simulink library "Copter_Library"  (Simulink 7.3)
settings: Solver=ode45  StartTime=0.0  StopTime=10.0  RelTol=1e-3
undefined symbols (not defined in the file or in its folder): boom, f1, f2, f3, f4, f5, g, I_x, I_y, I_z, m, speed, thrust, Ts
libraries: Copter_Library x10, dspinverses x2
settings Model: Creator=robert  LastModifiedBy=Alex

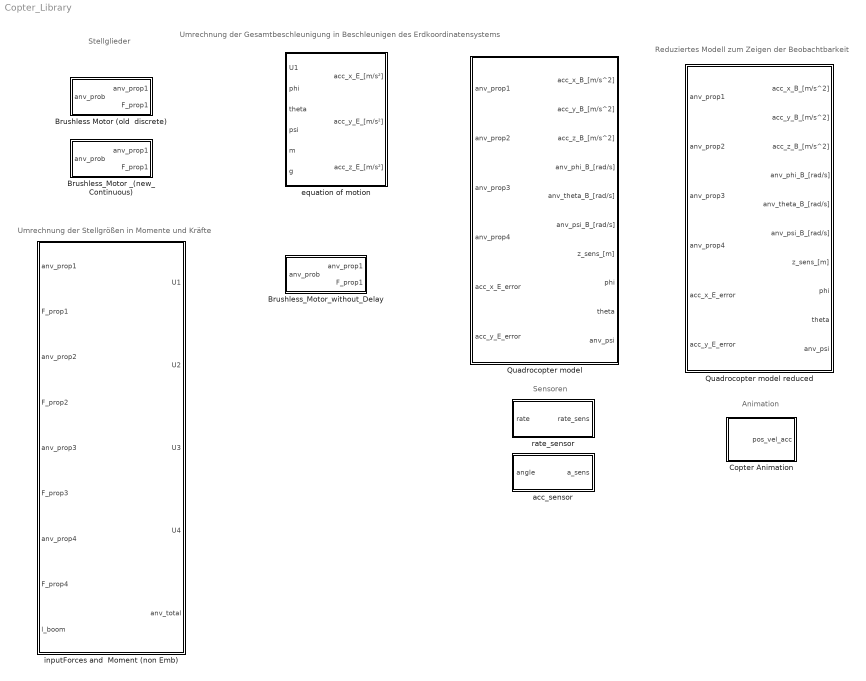
== system Copter_Library ==
  note: Sensoren
  note: Animation
  note: Umrechnung der Gesamtbeschleunigung in
      | Beschleunigen des Erdkoordinatensystems
  note: Stellglieder
  note: Umrechnung der Stellgrößen
      | in Momente und Kräfte
  note: Reduziertes Modell zum Zeigen der
      | Beobachtbarkeit
  Brushless Motor (old  discrete) : Subsystem
  Brushless_Motor _(new_Continuous) : Subsystem  mask{M_error=0.99}
      mask prompts: M_error "Motor-Force pitch error [1 = no error, 0.9 = 10% negativ error, 1.1 = 10% positive error]:"
  Brushless_Motor_without_Delay : Subsystem  AncestorBlock=Copter_Library/Brushless_Motor _(new_Continuous)  mask{M_error=0.99}
      mask prompts: M_error "Motor-Force pitch error [1 = no error, 0.9 = 10% negativ error, 1.1 = 10% positive error]:"
  Copter Animation : Subsystem  mask(Quadrocopter Animation){AXES=[-100 100 -100 100 0 100], T_INT=1/25, K_VAR=Feste Position, K_POS=[10 0 2], K_ANGLE=27, A_ON=on, u_phi=on, u_theta=on, u_psi=on, u_x=on, u_y=on, u_z=off}
      mask prompts: AXES "Achsen Grenzen [xmin xmax ymin ymax zmin zmax]"; T_INT "Zeitintervall zwischen Aktualisierungen [s]:"; K_VAR "Kamera Art:"; K_POS "Ort der Kamera [xc yc zc]:"; K_ANGLE "Öffnungswinkel der Kamera [Grad]:"; A_ON "Animation Einschalten:"; u_phi "Use Input phi:"; u_theta "Use Input theta:"; u_psi "Use Input psi:"; u_x "Use Input x:"; u_y "Use Input y:"; u_z "Use Input z:"
      mask help: Erstellt eine 3-D animierte Ansicht eines Quadrocopters.
      mask init:
      | Config.axes = AXES;
      | Config.update = T_INT;
      | Config.camera_view = K_VAR;
      | Config.camera_pos = K_POS;
      | Config.view = K_ANGLE;
      | Config.Animenable = A_ON;
      | Config.phi = u_phi;
      | Config.theta = u_theta;
      | Config.psi = u_psi;
      | Config.x = u_x;
      | Config.y = u_y;
      | Config.z = u_z;
      mask Help:
      | <p>Dieser Block erstellt ein 3 dimensionales Fenster eines Quadrocopters.
      | 
      | <p><H4>Block Eingänge</H4>
      | Der Eingangsvektor bestehend aus:
      | <ul>
      | <li>X-Koordinate - Ort bezogen auf die X-Achse
      | <li>Y-Koordinate - Ort bezogen auf die Y-Achse
      | <li>Z-Koordinate - Ort bezogen auf die Z-Achse
      | <li>Psi - Yaw Drehung um die Z-Achse
      | <li>Phi - Roll Drehen um die Achse in Flugrichtung
      | <li>theta - pitch Neigung in Flugrichtung nach oben bzw. unten
      | </ul></p>
      mask StyleString: edit,edit,popup(Feste Position|Frei bewegbar),edit,edit,checkbox,checkbox,checkbox,checkbox,checkbox,checkbox,checkbox
  Quadrocopter model : Subsystem
  Quadrocopter model reduced : Subsystem
  acc_sensor : Subsystem  mask{lsb_per_g=g/340, direction=1}
      mask prompts: lsb_per_g "Auflösung[LSB/g]:(g = Erdbeschleunigung)"; direction "Direction[-1 ... 1]:"
      mask init:
      | LSB_per_g = lsb_per_g;
      | Direction = direction;
  equation of motion : Subsystem
  inputForces and  Moment (non Emb) : Subsystem
  rate_sensor : Subsystem  mask{resolution=0.01423597337917052316100312926969, offset=505, direction=1}
      mask prompts: resolution "Resolution [(rad/sec)/LSB)]:"; offset "Offset [LSB]:"; direction "Direction [-1 ... 1]"
      mask init:
      | Resolution = resolution;
      | Offset = offset;
      | Direction = direction;

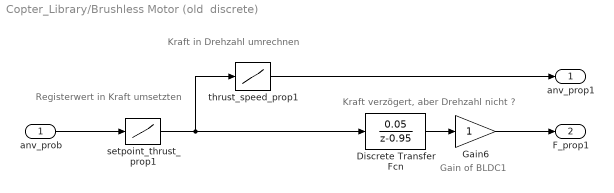
== system Copter_Library/Brushless Motor (old  discrete) ==
  note: Gain of BLDC1
  note: Kraft in Drehzahl umrechnen
  note: Registerwert in Kraft umsetzten
  note: Kraft verzögert, aber Drehzahl nicht ?
  anv_prob : Inport  OutDataType=fixdt(1, 16)  OutScaling=2^0
  Discrete Transfer Fcn : DiscreteTransferFcn  Numerator=[0.05]  Denominator=[1 -0.95]  SampleTime=Ts
  Gain6 : Gain  ParameterDataType=fixdt(1, 16)  ParameterScaling=2^0  OutDataType=fixdt(1, 16)  OutScaling=2^0
  setpoint_thrust_prop1 : Lookup  InputValues=[0 40 175]  Table=[0 500 4500]./1000  LookUpMeth=Interpolation-Use End Values  OutDataType=fixdt(1, 16)  OutScaling=2^0
  thrust_speed_prop1 : Lookup  InputValues=thrust  Table=speed  LookUpMeth=Interpolation-Use End Values  OutDataType=fixdt(1, 16)  OutScaling=2^0
  anv_prop1 : Outport  OutDataType=fixdt(1, 16)  OutScaling=2^0
  F_prop1 : Outport  Port=2  OutDataType=fixdt(1, 16)  OutScaling=2^0
  wires:
  anv_prob/1 -> setpoint_thrust_prop1/1
  Discrete Transfer Fcn/1 -> Gain6/1
  Gain6/1 -> F_prop1/1
  thrust_speed_prop1/1 -> anv_prop1/1
  setpoint_thrust_prop1/1 -> thrust_speed_prop1/1, Discrete Transfer Fcn/1

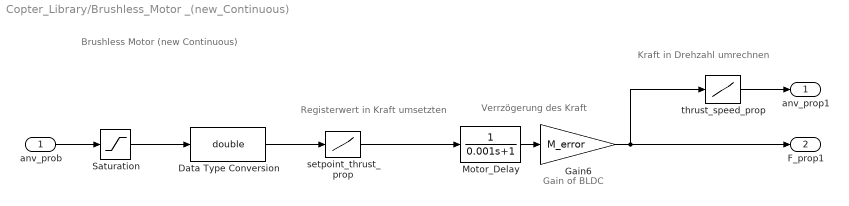
== system Copter_Library/Brushless_Motor _(new_Continuous) ==
  note: Gain of BLDC
  note: Kraft in Drehzahl umrechnen
  note: Registerwert in Kraft umsetzten
  note: Verrzögerung des Kraft
  note: Brushless Motor (new Continuous)
  anv_prob : Inport  OutDataType=fixdt(1, 16)  OutScaling=2^0
  Data Type Conversion : DataTypeConversion  OutDataTypeMode=double  OutDataType=fixdt(1, 16)  OutScaling=2^0  OutDataTypeStr=double
  Gain6 : Gain  Gain=M_error  ParameterDataType=fixdt(1, 16)  ParameterScaling=2^0  OutDataType=fixdt(1, 16)  OutScaling=2^0
  Motor_Delay : TransferFcn  Denominator=[0.001 1]  ContinuousStateAttributes='Motor_Delay'
  Saturation : Saturate  UpperLimit=255  LowerLimit=0  OutDataType=fixdt(1, 16)  OutScaling=2^0
  setpoint_thrust_prop : Lookup  InputValues=[0 40 175]  Table=[0 500 4500]./1000  LookUpMeth=Interpolation-Use End Values  OutDataType=fixdt(1, 16)  OutScaling=2^0
  thrust_speed_prop : Lookup  InputValues=thrust  Table=speed  LookUpMeth=Interpolation-Use End Values  OutDataType=fixdt(1, 16)  OutScaling=2^0
  anv_prop1 : Outport  OutDataType=fixdt(1, 16)  OutScaling=2^0
  F_prop1 : Outport  Port=2  OutDataType=fixdt(1, 16)  OutScaling=2^0
  wires:
  setpoint_thrust_prop/1 -> Motor_Delay/1
  Saturation/1 -> Data Type Conversion/1
  anv_prob/1 -> Saturation/1
  Data Type Conversion/1 -> setpoint_thrust_prop/1
  Motor_Delay/1 -> Gain6/1
  Gain6/1 -> F_prop1/1, thrust_speed_prop/1
  thrust_speed_prop/1 -> anv_prop1/1

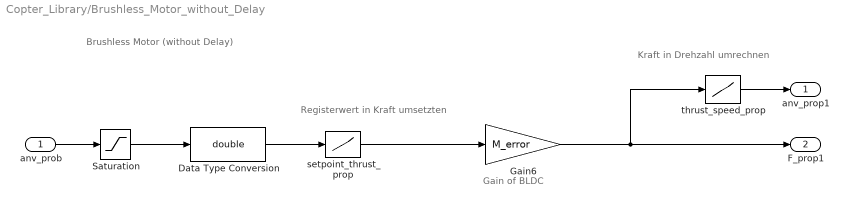
== system Copter_Library/Brushless_Motor_without_Delay ==
  note: Gain of BLDC
  note: Kraft in Drehzahl umrechnen
  note: Registerwert in Kraft umsetzten
  note: Brushless Motor (without Delay)
  anv_prob : Inport  OutDataType=fixdt(1, 16)  OutScaling=2^0
  Data Type Conversion : DataTypeConversion  OutDataTypeMode=double  OutDataType=fixdt(1, 16)  OutScaling=2^0  OutDataTypeStr=double
  Gain6 : Gain  Gain=M_error  ParameterDataType=fixdt(1, 16)  ParameterScaling=2^0  OutDataType=fixdt(1, 16)  OutScaling=2^0
  Saturation : Saturate  UpperLimit=255  LowerLimit=0  OutDataType=fixdt(1, 16)  OutScaling=2^0
  setpoint_thrust_prop : Lookup  InputValues=[0 40 175]  Table=[0 500 4500]./1000  LookUpMeth=Interpolation-Use End Values  OutDataType=fixdt(1, 16)  OutScaling=2^0
  thrust_speed_prop : Lookup  InputValues=thrust  Table=speed  LookUpMeth=Interpolation-Use End Values  OutDataType=fixdt(1, 16)  OutScaling=2^0
  anv_prop1 : Outport  OutDataType=fixdt(1, 16)  OutScaling=2^0
  F_prop1 : Outport  Port=2  OutDataType=fixdt(1, 16)  OutScaling=2^0
  wires:
  setpoint_thrust_prop/1 -> Gain6/1
  Saturation/1 -> Data Type Conversion/1
  anv_prob/1 -> Saturation/1
  Data Type Conversion/1 -> setpoint_thrust_prop/1
  Gain6/1 -> F_prop1/1, thrust_speed_prop/1
  thrust_speed_prop/1 -> anv_prop1/1

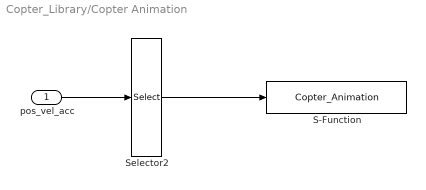
== system Copter_Library/Copter Animation ==
  pos_vel_acc : Inport  PortDimensions=19  OutDataType=sfix(16)  OutScaling=2^0
  S-Function : S-Function  FunctionName=Copter_Animation  Parameters=Config  EnableBusSupport=off
  Selector2 : Selector  InputPortWidth=19  IndexOptions=Index vector (dialog)  Indices=[1 2 3 4 5 6]  OutputSizes=1
  wires:
  Selector2/1 -> S-Function/1
  pos_vel_acc/1 -> Selector2/1

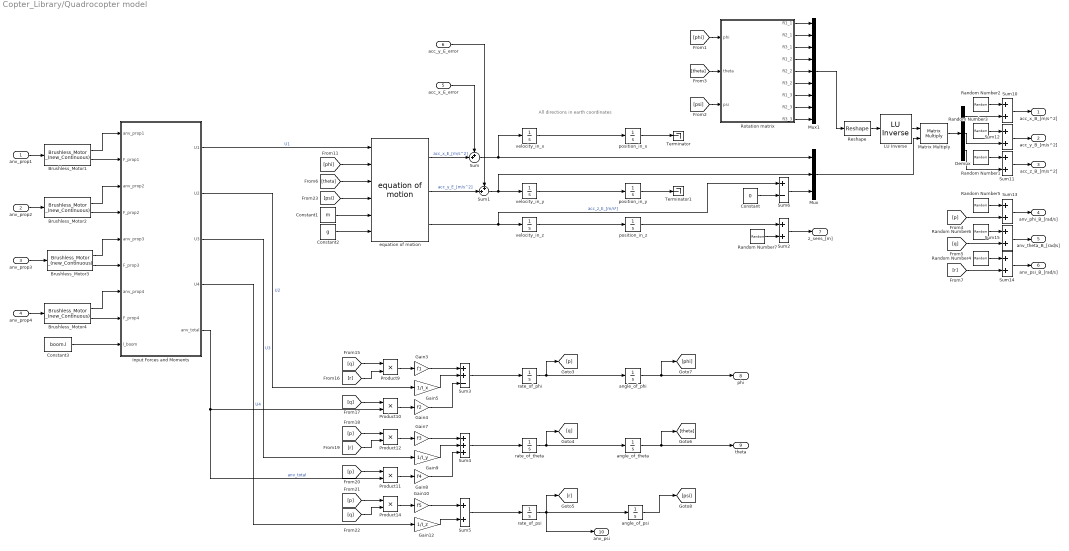
== system Copter_Library/Quadrocopter model ==
  note: All directions in earth coordinates
  anv_prop1 : Inport  OutDataType=fixdt(1, 16)  OutScaling=2^0
  anv_prop2 : Inport  Port=2  OutDataType=fixdt(1, 16)  OutScaling=2^0
  anv_prop3 : Inport  Port=3  OutDataType=fixdt(1, 16)  OutScaling=2^0
  anv_prop4 : Inport  Port=4  OutDataType=fixdt(1, 16)  OutScaling=2^0
  acc_x_E_error : Inport  Port=5  OutDataType=fixdt(1, 16)  OutScaling=2^0
  acc_y_E_error : Inport  Port=6  OutDataType=fixdt(1, 16)  OutScaling=2^0
  " LU Inverse" : dspinverses/ LU Inverse  SystemSampleTime=-1
  Brushless_Motor{1..4} (4 alike) : Copter_Library/Brushless_Motor _(new_Continuous)  SystemSampleTime=-1
  Constant : Constant  Value=0  OutDataType=fixdt(1, 16)  OutScaling=2^0  SampleTime=Ts
  Constant1 : Constant  Value=m  OutDataType=fixdt(1, 16)  OutScaling=2^0  SampleTime=Ts
  Constant2 : Constant  Value=g  OutDataType=fixdt(1, 16)  OutScaling=2^0  SampleTime=Ts
  Constant3 : Constant  Value=boom.l  OutDataType=fixdt(1, 16)  OutScaling=2^0
  Demux : Demux  Outputs=3
  Gain10 : Gain  Gain=f5  ParameterDataType=fixdt(1, 16)  ParameterScaling=2^0  OutDataType=fixdt(1, 16)  OutScaling=2^0
  Gain12 : Gain  Gain=1/I_z  ParameterDataType=fixdt(1, 16)  ParameterScaling=2^0  OutDataType=fixdt(1, 16)  OutScaling=2^0
  Gain3 : Gain  Gain=f1  ParameterDataType=fixdt(1, 16)  ParameterScaling=2^0  OutDataType=fixdt(1, 16)  OutScaling=2^0
  Gain4 : Gain  Gain=f2  ParameterDataType=fixdt(1, 16)  ParameterScaling=2^0  OutDataType=fixdt(1, 16)  OutScaling=2^0
  Gain5 : Gain  Gain=1/I_x  ParameterDataType=fixdt(1, 16)  ParameterScaling=2^0  OutDataType=fixdt(1, 16)  OutScaling=2^0
  Gain7 : Gain  Gain=f3  ParameterDataType=fixdt(1, 16)  ParameterScaling=2^0  OutDataType=fixdt(1, 16)  OutScaling=2^0
  Gain8 : Gain  Gain=f4  ParameterDataType=fixdt(1, 16)  ParameterScaling=2^0  OutDataType=fixdt(1, 16)  OutScaling=2^0
  Gain9 : Gain  Gain=1/I_y  ParameterDataType=fixdt(1, 16)  ParameterScaling=2^0  OutDataType=fixdt(1, 16)  OutScaling=2^0
  Input Forces and Moments : Stateflow chart
  Matrix Multiply : Product  Multiplication=Matrix(*)  OutDataType=sfix(16)  OutScaling=2^0
  Mux : Mux  Inputs=3
  Mux1 : Mux  Inputs=9
  Product{9..12,14} (5 alike) : Product  OutDataType=fixdt(1, 16)  OutScaling=2^0  RndMeth=Zero
  Random Number{1..7} (7 alike) : RandomNumber  Variance=0  SampleTime=Ts
  Reshape : Reshape  OutputDimensionality=Customize  OutputDimensions=[3,3]
  Rotation matrix : Stateflow chart
  Sum : Sum  Inputs=++|  OutDataType=fixdt(1, 16)  OutScaling=2^0
  Sum1 : Sum  Inputs=++|  OutDataType=fixdt(1, 16)  OutScaling=2^0
  Sum{2,5,10..15} (8 alike) : Sum  OutDataType=fixdt(1, 16)  OutScaling=2^0
  Sum3 : Sum  Inputs=++-  OutDataType=fixdt(1, 16)  OutScaling=2^0
  Sum4 : Sum  Inputs=+++  OutDataType=fixdt(1, 16)  OutScaling=2^0
  Sum6 : Sum  Inputs=+-  OutDataType=fixdt(1, 16)  OutScaling=2^0
  Terminator : Terminator
  Terminator1 : Terminator
  angle_of_phi : Integrator
  angle_of_psi : Integrator
  angle_of_theta : Integrator
  equation of motion : Copter_Library/equation of motion  SystemSampleTime=-1
  position_in_x : Integrator
  position_in_y : Integrator
  position_in_z : Integrator
  rate_of_phi : Integrator
  rate_of_psi : Integrator
  rate_of_theta : Integrator
  velocity_in_x : Integrator
  velocity_in_y : Integrator
  velocity_in_z : Integrator
  acc_x_B_[m/s^2] : Outport  OutDataType=fixdt(1, 16)  OutScaling=2^0
  acc_y_B_[m/s^2] : Outport  Port=2  OutDataType=fixdt(1, 16)  OutScaling=2^0
  acc_z_B_[m/s^2] : Outport  Port=3  OutDataType=fixdt(1, 16)  OutScaling=2^0
  anv_phi_B_[rad/s] : Outport  Port=4  OutDataType=fixdt(1, 16)  OutScaling=2^0
  anv_theta_B_[rad/s] : Outport  Port=5  OutDataType=fixdt(1, 16)  OutScaling=2^0
  anv_psi_B_[rad/s] : Outport  Port=6  OutDataType=fixdt(1, 16)  OutScaling=2^0
  z_sens_[m] : Outport  Port=7  OutDataType=fixdt(1, 16)  OutScaling=2^0
  phi : Outport  Port=8  OutDataType=fixdt(1, 16)  OutScaling=2^0
  theta : Outport  Port=9  OutDataType=fixdt(1, 16)  OutScaling=2^0
  anv_psi : Outport  Port=10  OutDataType=fixdt(1, 16)  OutScaling=2^0
  wires:
  Sum14/1 -> anv_psi_B_[rad/s]/1
  Sum15/1 -> anv_theta_B_[rad/s]/1
  Sum13/1 -> anv_phi_B_[rad/s]/1
  [q] -> Sum15/2
  Random Number6/1 -> Sum15/1
  [r] -> Sum14/2
  Random Number4/1 -> Sum14/1
  [p] -> Sum13/2
  Random Number5/1 -> Sum13/1
  Sum11/1 -> acc_z_B_[m/s^2]/1
  Sum12/1 -> acc_y_B_[m/s^2]/1
  Sum10/1 -> acc_x_B_[m/s^2]/1
  Demux/2 -> Sum12/2
  Random Number3/1 -> Sum12/1
  Demux/3 -> Sum11/2
  Random Number1/1 -> Sum11/1
  Demux/1 -> Sum10/2
  Random Number2/1 -> Sum10/1
  Matrix Multiply/1 -> Demux/1
  anv_prop3/1 -> Brushless_Motor3/1
  anv_prop4/1 -> Brushless_Motor4/1
  Reshape/1 -> " LU Inverse"/1
  Mux/1 -> Matrix Multiply/2
  Mux1/1 -> Reshape/1
  Rotation matrix/9(R3_3) -> Mux1/9
  Rotation matrix/8(R2_3) -> Mux1/8
  Rotation matrix/7(R1_3) -> Mux1/7
  Rotation matrix/6(R3_2) -> Mux1/6
  Rotation matrix/5(R2_2) -> Mux1/5
  Rotation matrix/4(R1_2) -> Mux1/4
  Rotation matrix/3(R3_1) -> Mux1/3
  Rotation matrix/2(R2_1) -> Mux1/2
  Rotation matrix/1(R1_1) -> Mux1/1
  [psi] -> Rotation matrix/3(psi)
  [theta] -> Rotation matrix/2(theta)
  [phi] -> Rotation matrix/1(phi)
  anv_prop2/1 -> Brushless_Motor2/1
  anv_prop1/1 -> Brushless_Motor1/1
  velocity_in_x/1 -> position_in_x/1
  velocity_in_y/1 -> position_in_y/1
  velocity_in_z/1 -> position_in_z/1
  Constant3/1 -> Input Forces and Moments/9(l_boom)
  Sum5/1 -> rate_of_psi/1
  Input Forces and Moments/4(U4) -> Gain12/1  "U4"
  Gain12/1 -> Sum5/2
  Gain10/1 -> Sum5/1
  Product14/1 -> Gain10/1
  [q] -> Product14/2
  [p] -> Product14/1
  Sum4/1 -> rate_of_theta/1
  Input Forces and Moments/3(U3) -> Gain9/1  "U3"
  Gain8/1 -> Sum4/3
  Gain9/1 -> Sum4/2
  Product11/1 -> Gain8/1
  [p] -> Product11/1
  Gain7/1 -> Sum4/1
  Product12/1 -> Gain7/1
  [r] -> Product12/2
  [p] -> Product12/1
  Input Forces and Moments/1(U1) -> equation of motion/1  "U1"
  Sum3/1 -> rate_of_phi/1
  Gain4/1 -> Sum3/3
  Gain5/1 -> Sum3/2
  Input Forces and Moments/2(U2) -> Gain5/1  "U2"
  Product10/1 -> Gain4/1
  [q] -> Product10/1
  Gain3/1 -> Sum3/1
  Product9/1 -> Gain3/1
  [r] -> Product9/2
  [q] -> Product9/1
  Input Forces and Moments/5(anv_total) -> Product11/2, Product10/2  "anv_total"
  angle_of_phi/1 -> [phi], phi/1
  angle_of_theta/1 -> [theta], theta/1
  angle_of_psi/1 -> [psi]
  rate_of_phi/1 -> [p], angle_of_phi/1
  rate_of_theta/1 -> angle_of_theta/1, [q]
  rate_of_psi/1 -> anv_psi/1, angle_of_psi/1, [r]
  Constant/1 -> Sum6/2
  Sum6/1 -> Mux/3
  " LU Inverse"/1 -> Matrix Multiply/1
  Brushless_Motor1/1 -> Input Forces and Moments/1(anv_prop1)
  Brushless_Motor1/2 -> Input Forces and Moments/2(F_prop1)
  Brushless_Motor2/1 -> Input Forces and Moments/3(anv_prop2)
  Brushless_Motor2/2 -> Input Forces and Moments/4(F_prop2)
  Brushless_Motor3/1 -> Input Forces and Moments/5(anv_prop3)
  Brushless_Motor3/2 -> Input Forces and Moments/6(F_prop3)
  Brushless_Motor4/1 -> Input Forces and Moments/7(anv_prop4)
  Brushless_Motor4/2 -> Input Forces and Moments/8(F_prop4)
  [phi] -> equation of motion/2
  [theta] -> equation of motion/3
  [psi] -> equation of motion/4
  Constant1/1 -> equation of motion/5
  Constant2/1 -> equation of motion/6
  equation of motion/3 -> velocity_in_z/1, Sum6/1  "acc_z_E_[m/s²]"
  position_in_x/1 -> Terminator/1
  position_in_y/1 -> Terminator1/1
  Sum1/1 -> velocity_in_y/1, Mux/2
  equation of motion/2 -> Sum1/2  "acc_y_E_[m/s^2]"
  equation of motion/1 -> Sum/2  "acc_x_E_[m/s^2]"
  Sum/1 -> Mux/1, velocity_in_x/1
  acc_x_E_error/1 -> Sum/1
  acc_y_E_error/1 -> Sum1/1
  position_in_z/1 -> Sum2/1
  Sum2/1 -> z_sens_[m]/1
  Random Number7/1 -> Sum2/2

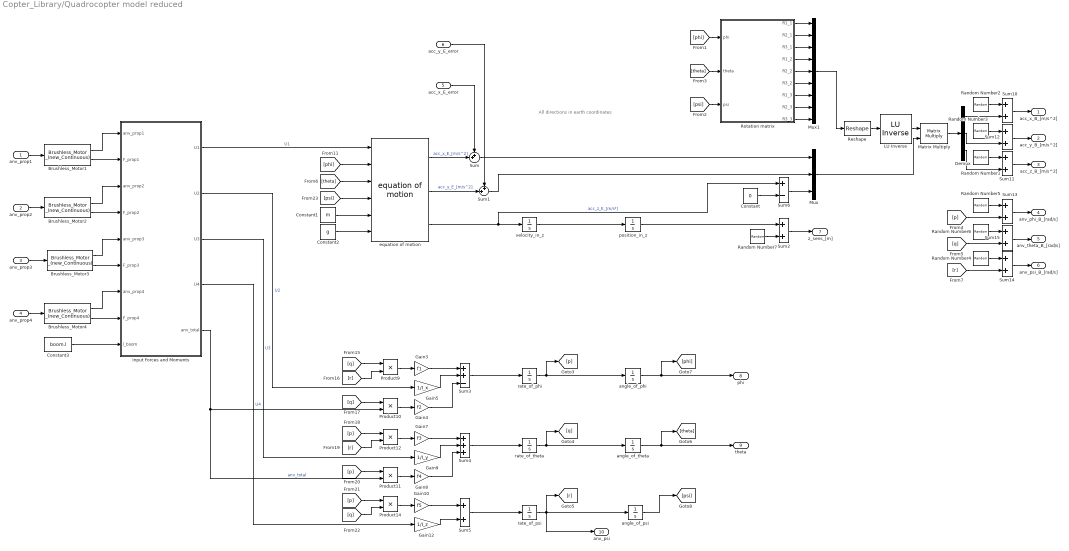
== system Copter_Library/Quadrocopter model reduced ==
  note: All directions in earth coordinates
  anv_prop1 : Inport  OutDataType=fixdt(1, 16)  OutScaling=2^0
  anv_prop2 : Inport  Port=2  OutDataType=fixdt(1, 16)  OutScaling=2^0
  anv_prop3 : Inport  Port=3  OutDataType=fixdt(1, 16)  OutScaling=2^0
  anv_prop4 : Inport  Port=4  OutDataType=fixdt(1, 16)  OutScaling=2^0
  acc_x_E_error : Inport  Port=5  OutDataType=fixdt(1, 16)  OutScaling=2^0
  acc_y_E_error : Inport  Port=6  OutDataType=fixdt(1, 16)  OutScaling=2^0
  " LU Inverse" : dspinverses/ LU Inverse  SystemSampleTime=-1
  Brushless_Motor{1..4} (4 alike) : Copter_Library/Brushless_Motor _(new_Continuous)  SystemSampleTime=-1
  Constant : Constant  Value=0  OutDataType=fixdt(1, 16)  OutScaling=2^0  SampleTime=Ts
  Constant1 : Constant  Value=m  OutDataType=fixdt(1, 16)  OutScaling=2^0  SampleTime=Ts
  Constant2 : Constant  Value=g  OutDataType=fixdt(1, 16)  OutScaling=2^0  SampleTime=Ts
  Constant3 : Constant  Value=boom.l  OutDataType=fixdt(1, 16)  OutScaling=2^0
  Demux : Demux  Outputs=3
  Gain10 : Gain  Gain=f5  ParameterDataType=fixdt(1, 16)  ParameterScaling=2^0  OutDataType=fixdt(1, 16)  OutScaling=2^0
  Gain12 : Gain  Gain=1/I_z  ParameterDataType=fixdt(1, 16)  ParameterScaling=2^0  OutDataType=fixdt(1, 16)  OutScaling=2^0
  Gain3 : Gain  Gain=f1  ParameterDataType=fixdt(1, 16)  ParameterScaling=2^0  OutDataType=fixdt(1, 16)  OutScaling=2^0
  Gain4 : Gain  Gain=f2  ParameterDataType=fixdt(1, 16)  ParameterScaling=2^0  OutDataType=fixdt(1, 16)  OutScaling=2^0
  Gain5 : Gain  Gain=1/I_x  ParameterDataType=fixdt(1, 16)  ParameterScaling=2^0  OutDataType=fixdt(1, 16)  OutScaling=2^0
  Gain7 : Gain  Gain=f3  ParameterDataType=fixdt(1, 16)  ParameterScaling=2^0  OutDataType=fixdt(1, 16)  OutScaling=2^0
  Gain8 : Gain  Gain=f4  ParameterDataType=fixdt(1, 16)  ParameterScaling=2^0  OutDataType=fixdt(1, 16)  OutScaling=2^0
  Gain9 : Gain  Gain=1/I_y  ParameterDataType=fixdt(1, 16)  ParameterScaling=2^0  OutDataType=fixdt(1, 16)  OutScaling=2^0
  Input Forces and Moments : Stateflow chart
  Matrix Multiply : Product  Multiplication=Matrix(*)  OutDataType=sfix(16)  OutScaling=2^0
  Mux : Mux  Inputs=3
  Mux1 : Mux  Inputs=9
  Product{9..12,14} (5 alike) : Product  OutDataType=fixdt(1, 16)  OutScaling=2^0  RndMeth=Zero
  Random Number{1..7} (7 alike) : RandomNumber  Variance=0  SampleTime=Ts
  Reshape : Reshape  OutputDimensionality=Customize  OutputDimensions=[3,3]
  Rotation matrix : Stateflow chart
  Sum : Sum  Inputs=++|  OutDataType=fixdt(1, 16)  OutScaling=2^0
  Sum1 : Sum  Inputs=++|  OutDataType=fixdt(1, 16)  OutScaling=2^0
  Sum{2,5,10..15} (8 alike) : Sum  OutDataType=fixdt(1, 16)  OutScaling=2^0
  Sum3 : Sum  Inputs=++-  OutDataType=fixdt(1, 16)  OutScaling=2^0
  Sum4 : Sum  Inputs=+++  OutDataType=fixdt(1, 16)  OutScaling=2^0
  Sum6 : Sum  Inputs=+-  OutDataType=fixdt(1, 16)  OutScaling=2^0
  angle_of_phi : Integrator
  angle_of_psi : Integrator
  angle_of_theta : Integrator
  equation of motion : Copter_Library/equation of motion  SystemSampleTime=-1
  position_in_z : Integrator
  rate_of_phi : Integrator
  rate_of_psi : Integrator
  rate_of_theta : Integrator
  velocity_in_z : Integrator
  acc_x_B_[m/s^2] : Outport  OutDataType=fixdt(1, 16)  OutScaling=2^0
  acc_y_B_[m/s^2] : Outport  Port=2  OutDataType=fixdt(1, 16)  OutScaling=2^0
  acc_z_B_[m/s^2] : Outport  Port=3  OutDataType=fixdt(1, 16)  OutScaling=2^0
  anv_phi_B_[rad/s] : Outport  Port=4  OutDataType=fixdt(1, 16)  OutScaling=2^0
  anv_theta_B_[rad/s] : Outport  Port=5  OutDataType=fixdt(1, 16)  OutScaling=2^0
  anv_psi_B_[rad/s] : Outport  Port=6  OutDataType=fixdt(1, 16)  OutScaling=2^0
  z_sens_[m] : Outport  Port=7  OutDataType=fixdt(1, 16)  OutScaling=2^0
  phi : Outport  Port=8  OutDataType=fixdt(1, 16)  OutScaling=2^0
  theta : Outport  Port=9  OutDataType=fixdt(1, 16)  OutScaling=2^0
  anv_psi : Outport  Port=10  OutDataType=fixdt(1, 16)  OutScaling=2^0
  wires:
  Sum14/1 -> anv_psi_B_[rad/s]/1
  Sum15/1 -> anv_theta_B_[rad/s]/1
  Sum13/1 -> anv_phi_B_[rad/s]/1
  [q] -> Sum15/2
  Random Number6/1 -> Sum15/1
  [r] -> Sum14/2
  Random Number4/1 -> Sum14/1
  [p] -> Sum13/2
  Random Number5/1 -> Sum13/1
  Sum11/1 -> acc_z_B_[m/s^2]/1
  Sum12/1 -> acc_y_B_[m/s^2]/1
  Sum10/1 -> acc_x_B_[m/s^2]/1
  Demux/2 -> Sum12/2
  Random Number3/1 -> Sum12/1
  Demux/3 -> Sum11/2
  Random Number1/1 -> Sum11/1
  Demux/1 -> Sum10/2
  Random Number2/1 -> Sum10/1
  Matrix Multiply/1 -> Demux/1
  anv_prop3/1 -> Brushless_Motor3/1
  anv_prop4/1 -> Brushless_Motor4/1
  Reshape/1 -> " LU Inverse"/1
  Mux/1 -> Matrix Multiply/2
  Mux1/1 -> Reshape/1
  Rotation matrix/9(R3_3) -> Mux1/9
  Rotation matrix/8(R2_3) -> Mux1/8
  Rotation matrix/7(R1_3) -> Mux1/7
  Rotation matrix/6(R3_2) -> Mux1/6
  Rotation matrix/5(R2_2) -> Mux1/5
  Rotation matrix/4(R1_2) -> Mux1/4
  Rotation matrix/3(R3_1) -> Mux1/3
  Rotation matrix/2(R2_1) -> Mux1/2
  Rotation matrix/1(R1_1) -> Mux1/1
  [psi] -> Rotation matrix/3(psi)
  [theta] -> Rotation matrix/2(theta)
  [phi] -> Rotation matrix/1(phi)
  anv_prop2/1 -> Brushless_Motor2/1
  anv_prop1/1 -> Brushless_Motor1/1
  velocity_in_z/1 -> position_in_z/1
  Constant3/1 -> Input Forces and Moments/9(l_boom)
  Sum5/1 -> rate_of_psi/1
  Input Forces and Moments/4(U4) -> Gain12/1  "U4"
  Gain12/1 -> Sum5/2
  Gain10/1 -> Sum5/1
  Product14/1 -> Gain10/1
  [q] -> Product14/2
  [p] -> Product14/1
  Sum4/1 -> rate_of_theta/1
  Input Forces and Moments/3(U3) -> Gain9/1  "U3"
  Gain8/1 -> Sum4/3
  Gain9/1 -> Sum4/2
  Product11/1 -> Gain8/1
  [p] -> Product11/1
  Gain7/1 -> Sum4/1
  Product12/1 -> Gain7/1
  [r] -> Product12/2
  [p] -> Product12/1
  Input Forces and Moments/1(U1) -> equation of motion/1  "U1"
  Sum3/1 -> rate_of_phi/1
  Gain4/1 -> Sum3/3
  Gain5/1 -> Sum3/2
  Input Forces and Moments/2(U2) -> Gain5/1  "U2"
  Product10/1 -> Gain4/1
  [q] -> Product10/1
  Gain3/1 -> Sum3/1
  Product9/1 -> Gain3/1
  [r] -> Product9/2
  [q] -> Product9/1
  Input Forces and Moments/5(anv_total) -> Product11/2, Product10/2  "anv_total"
  angle_of_phi/1 -> [phi], phi/1
  angle_of_theta/1 -> [theta], theta/1
  angle_of_psi/1 -> [psi]
  rate_of_phi/1 -> [p], angle_of_phi/1
  rate_of_theta/1 -> angle_of_theta/1, [q]
  rate_of_psi/1 -> anv_psi/1, angle_of_psi/1, [r]
  Constant/1 -> Sum6/2
  Sum6/1 -> Mux/3
  " LU Inverse"/1 -> Matrix Multiply/1
  Brushless_Motor1/1 -> Input Forces and Moments/1(anv_prop1)
  Brushless_Motor1/2 -> Input Forces and Moments/2(F_prop1)
  Brushless_Motor2/1 -> Input Forces and Moments/3(anv_prop2)
  Brushless_Motor2/2 -> Input Forces and Moments/4(F_prop2)
  Brushless_Motor3/1 -> Input Forces and Moments/5(anv_prop3)
  Brushless_Motor3/2 -> Input Forces and Moments/6(F_prop3)
  Brushless_Motor4/1 -> Input Forces and Moments/7(anv_prop4)
  Brushless_Motor4/2 -> Input Forces and Moments/8(F_prop4)
  [phi] -> equation of motion/2
  [theta] -> equation of motion/3
  [psi] -> equation of motion/4
  Constant1/1 -> equation of motion/5
  Constant2/1 -> equation of motion/6
  equation of motion/3 -> velocity_in_z/1, Sum6/1  "acc_z_E_[m/s²]"
  Sum1/1 -> Mux/2
  equation of motion/2 -> Sum1/2  "acc_y_E_[m/s^2]"
  equation of motion/1 -> Sum/2  "acc_x_E_[m/s^2]"
  Sum/1 -> Mux/1
  acc_x_E_error/1 -> Sum/1
  acc_y_E_error/1 -> Sum1/1
  position_in_z/1 -> Sum2/1
  Sum2/1 -> z_sens_[m]/1
  Random Number7/1 -> Sum2/2

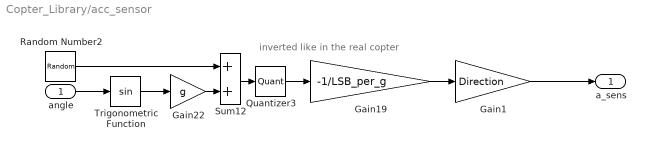
== system Copter_Library/acc_sensor ==
  note: inverted like in the real copter
  angle : Inport  OutDataType=fixdt(1, 16)  OutScaling=2^0
  Gain1 : Gain  Gain=Direction  ParameterDataType=fixdt(1, 16)  ParameterScaling=2^0  OutDataType=fixdt(1, 16)  OutScaling=2^0
  Gain19 : Gain  Gain=-1/LSB_per_g  ParameterDataType=fixdt(1, 16)  ParameterScaling=2^0  OutDataType=fixdt(1, 16)  OutScaling=2^0
  Gain22 : Gain  Gain=g  ParameterDataType=fixdt(1, 16)  ParameterScaling=2^0  OutDataType=fixdt(1, 16)  OutScaling=2^0
  Quantizer3 : Quantizer  QuantizationInterval=LSB_per_g  SampleTime=Ts
  Random Number2 : RandomNumber  Variance=0.0003  Seed=4564  SampleTime=0.01
  Sum12 : Sum  OutDataType=fixdt(1, 16)  OutScaling=2^0
  Trigonometric Function : Trigonometry
  a_sens : Outport  OutDataType=fixdt(1, 16)  OutScaling=2^0
  wires:
  Random Number2/1 -> Sum12/1
  Sum12/1 -> Quantizer3/1
  Trigonometric Function/1 -> Gain22/1
  Gain22/1 -> Sum12/2
  Quantizer3/1 -> Gain19/1
  angle/1 -> Trigonometric Function/1
  Gain19/1 -> Gain1/1
  Gain1/1 -> a_sens/1

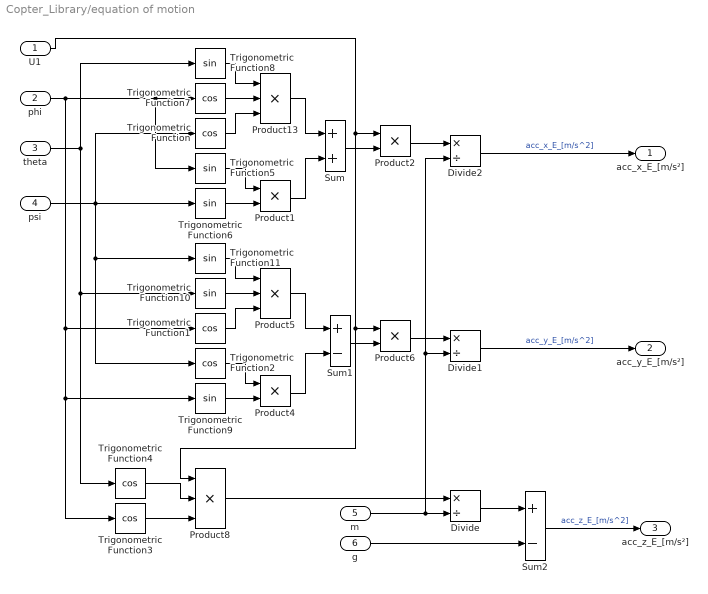
== system Copter_Library/equation of motion ==
  U1 : Inport  OutDataType=fixdt(1, 16)  OutScaling=2^0
  phi : Inport  Port=2  OutDataType=fixdt(1, 16)  OutScaling=2^0
  theta : Inport  Port=3  OutDataType=fixdt(1, 16)  OutScaling=2^0
  psi : Inport  Port=4  OutDataType=fixdt(1, 16)  OutScaling=2^0
  m : Inport  Port=5  OutDataType=fixdt(1, 16)  OutScaling=2^0
  g : Inport  Port=6  OutDataType=fixdt(1, 16)  OutScaling=2^0
  Divide : Product  Inputs=*/  OutDataType=fixdt(1, 16)  OutScaling=2^-10
  Divide1 : Product  Inputs=*/  OutDataType=fixdt(1, 16)  OutScaling=2^-10
  Divide2 : Product  Inputs=*/  OutDataType=fixdt(1, 16)  OutScaling=2^-10
  Product{1..2,4,6} (4 alike) : Product  OutDataType=fixdt(1, 16)  OutScaling=2^0  RndMeth=Zero
  Product13 : Product  Inputs=3  OutDataType=fixdt(1, 16)  OutScaling=2^0  RndMeth=Zero
  Product5 : Product  Inputs=3  OutDataType=fixdt(1, 16)  OutScaling=2^0  RndMeth=Zero
  Product8 : Product  Inputs=3  OutDataType=fixdt(1, 16)  OutScaling=2^0  RndMeth=Zero
  Sum : Sum  OutDataType=fixdt(1, 16)  OutScaling=2^0
  Sum1 : Sum  Inputs=+-  OutDataType=fixdt(1, 16)  OutScaling=2^0
  Sum2 : Sum  Inputs=+-  OutDataType=fixdt(1, 16)  OutScaling=2^0
  Trigonometric Function{,1..4,7} (6 alike) : Trigonometry  Operator=cos
  Trigonometric Function{5..6,8..11} (6 alike) : Trigonometry
  acc_x_E_[m/s²] : Outport  OutDataType=fixdt(1, 16)  OutScaling=2^0
  acc_y_E_[m/s²] : Outport  Port=2  OutDataType=fixdt(1, 16)  OutScaling=2^0
  acc_z_E_[m/s²] : Outport  Port=3  OutDataType=fixdt(1, 16)  OutScaling=2^0
  wires:
  g/1 -> Sum2/2
  Trigonometric Function4/1 -> Product8/2
  Trigonometric Function3/1 -> Product8/3
  Divide/1 -> Sum2/1
  Divide2/1 -> acc_x_E_[m/s²]/1  "acc_x_E_[m/s^2]"
  Product6/1 -> Divide1/1
  Sum1/1 -> Product6/2
  Product5/1 -> Sum1/1
  Trigonometric Function1/1 -> Product5/3
  Trigonometric Function10/1 -> Product5/2
  Trigonometric Function11/1 -> Product5/1
  Product4/1 -> Sum1/2
  Trigonometric Function2/1 -> Product4/1
  Trigonometric Function9/1 -> Product4/2
  Product2/1 -> Divide2/1
  Sum/1 -> Product2/2
  Product13/1 -> Sum/1
  Trigonometric Function/1 -> Product13/3
  Trigonometric Function7/1 -> Product13/2
  Trigonometric Function8/1 -> Product13/1
  Product1/1 -> Sum/2
  Trigonometric Function5/1 -> Product1/1
  Trigonometric Function6/1 -> Product1/2
  psi/1 -> Trigonometric Function2/1, Trigonometric Function11/1, Trigonometric Function/1, Trigonometric Function6/1
  theta/1 -> Trigonometric Function10/1, Trigonometric Function4/1, Trigonometric Function8/1
  Divide1/1 -> acc_y_E_[m/s²]/1  "acc_y_E_[m/s^2]"
  phi/1 -> Trigonometric Function9/1, Trigonometric Function3/1, Trigonometric Function1/1, Trigonometric Function7/1, Trigonometric Function5/1
  Product8/1 -> Divide/1
  U1/1 -> Product8/1, Product6/1, Product2/1
  m/1 -> Divide/2, Divide1/2, Divide2/2
  Sum2/1 -> acc_z_E_[m/s²]/1  "acc_z_E_[m/s^2]"

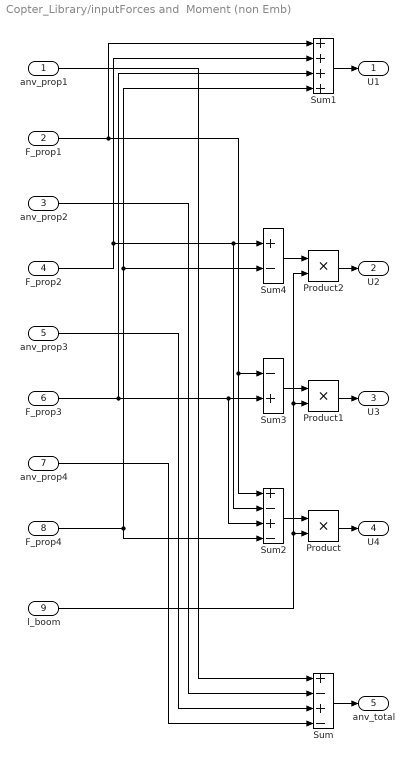
== system Copter_Library/inputForces and  Moment (non Emb) ==
  anv_prop1 : Inport  OutDataType=fixdt(1, 16)  OutScaling=2^0
  F_prop1 : Inport  Port=2  OutDataType=fixdt(1, 16)  OutScaling=2^0
  anv_prop2 : Inport  Port=3  OutDataType=fixdt(1, 16)  OutScaling=2^0
  F_prop2 : Inport  Port=4  OutDataType=fixdt(1, 16)  OutScaling=2^0
  anv_prop3 : Inport  Port=5  OutDataType=fixdt(1, 16)  OutScaling=2^0
  F_prop3 : Inport  Port=6  OutDataType=fixdt(1, 16)  OutScaling=2^0
  anv_prop4 : Inport  Port=7  OutDataType=fixdt(1, 16)  OutScaling=2^0
  F_prop4 : Inport  Port=8  OutDataType=fixdt(1, 16)  OutScaling=2^0
  l_boom : Inport  Port=9  OutDataType=fixdt(1, 16)  OutScaling=2^0
  Product : Product  OutDataType=fixdt(1, 16)  OutScaling=2^0  RndMeth=Zero
  Product1 : Product  OutDataType=fixdt(1, 16)  OutScaling=2^0  RndMeth=Zero
  Product2 : Product  OutDataType=fixdt(1, 16)  OutScaling=2^0  RndMeth=Zero
  Sum : Sum  Inputs=+-+-  OutDataType=fixdt(1, 16)  OutScaling=2^0
  Sum1 : Sum  Inputs=++++  OutDataType=fixdt(1, 16)  OutScaling=2^0
  Sum2 : Sum  Inputs=+-+-  OutDataType=fixdt(1, 16)  OutScaling=2^0
  Sum3 : Sum  Inputs=-+  OutDataType=fixdt(1, 16)  OutScaling=2^0
  Sum4 : Sum  Inputs=+-  OutDataType=fixdt(1, 16)  OutScaling=2^0
  U1 : Outport  OutDataType=fixdt(1, 16)  OutScaling=2^0
  U2 : Outport  Port=2  OutDataType=fixdt(1, 16)  OutScaling=2^0
  U3 : Outport  Port=3  OutDataType=fixdt(1, 16)  OutScaling=2^0
  U4 : Outport  Port=4  OutDataType=fixdt(1, 16)  OutScaling=2^0
  anv_total : Outport  Port=5  OutDataType=fixdt(1, 16)  OutScaling=2^0
  wires:
  Sum/1 -> anv_total/1
  anv_prop4/1 -> Sum/4
  anv_prop3/1 -> Sum/3
  anv_prop2/1 -> Sum/2
  anv_prop1/1 -> Sum/1
  Sum1/1 -> U1/1
  F_prop1/1 -> Sum1/1, Sum3/1, Sum2/1
  F_prop2/1 -> Sum1/2, Sum4/1, Sum2/2
  F_prop3/1 -> Sum1/3, Sum3/2, Sum2/3
  F_prop4/1 -> Sum1/4, Sum4/2, Sum2/4
  l_boom/1 -> Product/2, Product1/2, Product2/2
  Sum4/1 -> Product2/1
  Sum3/1 -> Product1/1
  Sum2/1 -> Product/1
  Product2/1 -> U2/1
  Product1/1 -> U3/1
  Product/1 -> U4/1

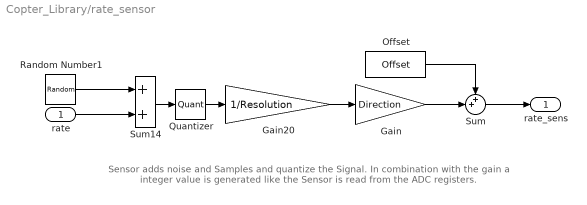
== system Copter_Library/rate_sensor ==
  note: Sensor adds noise and Samples and quantize the Signal. In combination with the gain a integer value is generated
      | like the Sensor is read from the ADC registers.
  rate : Inport  OutDataType=fixdt(1, 16)  OutScaling=2^0
  Gain : Gain  Gain=Direction  ParameterDataType=fixdt(1, 16)  ParameterScaling=2^0  OutDataType=fixdt(1, 16)  OutScaling=2^0
  Gain20 : Gain  Gain=1/Resolution  ParameterDataType=fixdt(1, 16)  ParameterScaling=2^0  OutDataType=fixdt(1, 16)  OutScaling=2^0
  Offset : Constant  Value=Offset  OutDataType=fixdt(1, 16)  OutScaling=2^0
  Quantizer : Quantizer  QuantizationInterval=Resolution  SampleTime=Ts
  Random Number1 : RandomNumber  Variance=3.0462e-8  Seed=45632  SampleTime=0.01
  Sum : Sum  Inputs=++|  OutDataType=fixdt(1, 16)  OutScaling=2^0
  Sum14 : Sum  OutDataType=fixdt(1, 16)  OutScaling=2^0
  rate_sens : Outport  OutDataType=fixdt(1, 16)  OutScaling=2^0
  wires:
  Random Number1/1 -> Sum14/1
  Sum14/1 -> Quantizer/1
  Quantizer/1 -> Gain20/1
  rate/1 -> Sum14/2
  Offset/1 -> Sum/1
  Sum/1 -> rate_sens/1
  Gain20/1 -> Gain/1
  Gain/1 -> Sum/2

== matlab function Quadrocopter model/Input Forces and Moments ==
  data: anv_prop1 input double; F_prop1 input double; anv_prop2 input double; F_prop2 input double; anv_prop3 input double; F_prop3 input double; anv_prop4 input double; U1 output double; F_prop4 input double; U2 output double; U3 output double; U4 output double; l_boom input double; anv_total output double
function [U1, U2, U3, U4, anv_total] = input(anv_prop1,F_prop1,anv_prop2,...
    F_prop2,anv_prop3,F_prop3,anv_prop4,F_prop4,l_boom)
%#eml

% Calculating Thrust in z-axis with respect to body fixed coordinate system
U1 = F_prop1 + F_prop2 + F_prop3 + F_prop4;             % [N]

% Calculating Torque around x-axis (Roll) due to Thrust
U2 = l_boom*(-F_prop4+F_prop2);                         % [Nm]

% Calculating Torque around y-axis (Pitch) due to Thrust
U3 = l_boom*(-F_prop1+F_prop3);                         % [Nm]

% Calculating Torque around z-axis (Yaw) due to Thrust
U4 = l_boom*(F_prop1-F_prop2+F_prop3-F_prop4);          % [Nm]

% Overall propeller speed
anv_total = anv_prop1-anv_prop2+anv_prop3-anv_prop4;    % [rad/s]

== matlab function Quadrocopter model/Rotation matrix ==
  data: phi input double; theta input double; psi input double; R1_1 output double; R2_1 output double; R3_1 output double; R1_2 output double; R2_2 output double; R3_2 output double; R1_3 output double; R2_3 output double; R3_3 output double
function [ R1_1, R2_1, R3_1, R1_2, R2_2, R3_2, R1_3, R2_3, R3_3] = input...
                                                    (phi, theta, psi)
% Transformation of E-frame to B-Frame
R1_1 = cos(psi)*cos(theta);
R2_1 = sin(psi)*cos(theta);
R3_1 = -sin(theta);
R1_2 = -sin(psi)*cos(phi)+cos(psi)*sin(theta)*sin(phi);
R2_2 = cos(psi)*cos(phi)+sin(psi)*sin(theta)*sin(phi);
R3_2 = cos(theta)*sin(phi);
R1_3 = sin(psi)*sin(phi)+cos(psi)*sin(theta)*cos(phi);
R2_3 = -cos(psi)*sin(phi)+sin(psi)*sin(theta)*cos(phi);
R3_3 = cos(theta)*cos(phi);

== matlab function Quadrocopter model reduced/Input Forces and Moments ==
  data: anv_prop1 input double; F_prop1 input double; anv_prop2 input double; F_prop2 input double; anv_prop3 input double; F_prop3 input double; anv_prop4 input double; U1 output double; F_prop4 input double; U2 output double; U3 output double; U4 output double; l_boom input double; anv_total output double
function [U1, U2, U3, U4, anv_total] = input(anv_prop1,F_prop1,anv_prop2,...
    F_prop2,anv_prop3,F_prop3,anv_prop4,F_prop4,l_boom)
%#eml

% Calculating Thrust in z-axis with respect to body fixed coordinate system
U1 = F_prop1 + F_prop2 + F_prop3 + F_prop4;             % [N]

% Calculating Torque around x-axis (Roll) due to Thrust
U2 = l_boom*(-F_prop4+F_prop2);                         % [Nm]

% Calculating Torque around y-axis (Pitch) due to Thrust
U3 = l_boom*(-F_prop1+F_prop3);                         % [Nm]

% Calculating Torque around z-axis (Yaw) due to Thrust
U4 = l_boom*(F_prop1-F_prop2+F_prop3-F_prop4);          % [Nm]

% Overall propeller speed
anv_total = anv_prop1-anv_prop2+anv_prop3-anv_prop4;    % [rad/s]

== matlab function Quadrocopter model reduced/Rotation matrix ==
  data: phi input double; theta input double; psi input double; R1_1 output double; R2_1 output double; R3_1 output double; R1_2 output double; R2_2 output double; R3_2 output double; R1_3 output double; R2_3 output double; R3_3 output double
function [ R1_1, R2_1, R3_1, R1_2, R2_2, R3_2, R1_3, R2_3, R3_3] = input...
                                                    (phi, theta, psi)
% Transformation of E-frame to B-Frame
R1_1 = cos(psi)*cos(theta);
R2_1 = sin(psi)*cos(theta);
R3_1 = -sin(theta);
R1_2 = -sin(psi)*cos(phi)+cos(psi)*sin(theta)*sin(phi);
R2_2 = cos(psi)*cos(phi)+sin(psi)*sin(theta)*sin(phi);
R3_2 = cos(theta)*sin(phi);
R1_3 = sin(psi)*sin(phi)+cos(psi)*sin(theta)*cos(phi);
R2_3 = -cos(psi)*sin(phi)+sin(psi)*sin(theta)*cos(phi);
R3_3 = cos(theta)*cos(phi);
